simulink model "sim1"  (R2023b)
settings: Solver=VariableStepAuto  StartTime=0.0  StopTime=0.05  RelTol=1e-3
settings Model: Creator=denismatveev  LastModifiedBy=denismatveev

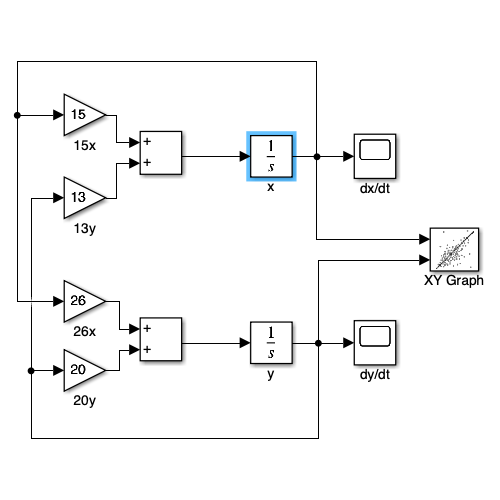
[thumbnail: Simulink's stored preview of the top-level diagram]
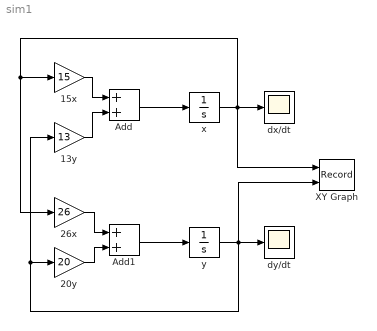
== system sim1 ==
  13y : Gain  Gain=13
  15x : Gain  Gain=15
  20y : Gain  Gain=20
  26x : Gain  Gain=26
  Add : Sum
  Add1 : Sum
  XY Graph : Record  FileSettingsInternal="{\"entries\":[{\"content\":{\"excelSettings\":{\"content\":{},\"type\":\"Streamout.ExcelSettings\"}},\"type\":\"Streamout.FileSettingStorage\",\"uuid\":\"\"}],\"packageUris\":[\"http:\\/\\/schema.mathworks.com\\/mf0\\/streamout_blocks\\/R2020a\"],\"version\":\"1.0\"}"  Layout=[1 1]  SignalsInternal="{\"entries\":[{\"content\":{\"signals\":[{\"content\":{\"blockPath\":[],\"dimensions\":[1],\"domain\":\"\",\"lineColor\":\"#a2142f\",\"lineWidth\":4,\"plots\":[1],\"port\":1,\"sid\":[\"\"],\"signalID\":2252,\"signalName\":\"x\"},\"type\":\"RecordBlkView.Signal\",\"uuid\":\"\"},{\"content\":{\"blockPath\":[],\"dimensions\":[1],\"domain\":\"\",\"lineColor\":\"#139fff\",\"plots\":[1],\"port\":2,\"sid\":[\"\"],\"signalID\":2256,\"signalName\":\"y\"},\"type\":\"RecordBlkView.Signal\",\"uuid\":\"\"}]},\"type\":\"RecordBlkView.InputSignals\",\"uuid\":\"\"}],\"packageUris\":[\"http:\\/\\/schema.mathworks.com\\/mf0\\/streamout_blocks\\/R2020a\"],\"version\":\"1.0\"}"  VisualizationBindings="{\"xyplotplugin\":{\"info\":[{\"series\":[{\"bindingParametersList\":[{\"parameter\":\"X-Axis\",\"signalID\":2252,\"signalName\":\"x\"},{\"parameter\":\"Y-Axis\",\"signalID\":2256,\"signalName\":\"y\"}],\"seriesID\":58494}],\"subplotID\":1}]}}"  CompatibilityTag=XY
  dx/dt : Scope
  dy/dt : Scope
  x : Integrator  InitialCondition=-10
  y : Integrator  InitialCondition=-10
  wires:
  15x/1 -> Add/1
  13y/1 -> Add/2
  Add/1 -> x/1
  x/1 -> XY Graph/1, dx/dt/1, 15x/1, 26x/1
  y/1 -> XY Graph/2, dy/dt/1, 13y/1, 20y/1
  26x/1 -> Add1/1
  20y/1 -> Add1/2
  Add1/1 -> y/1
